simulink model "softmax_int"  (R2024b)
settings: Solver=FixedStepDiscrete  StartTime=0.0  StopTime=20.0  RelTol=1e-3
InitFcn:
  | % Define a random matrix size between 3 and 10
  | n =6;
  | 
  | fprintf('Size of matrix A: n = %d\n', n);
libraries: simulink x1
settings Model: DataTypeOverride=Off  Creator=valen  LastModifiedBy=valen
settings SolverCC: AlgebraicLoopSolver=TrustRegion
settings DataIOCC: LimitDataPoints=on  SaveOutput=off  SaveTime=off
settings OptimizationCC: BlockReduction=off  ConditionallyExecuteInputs=off  DefaultParameterBehavior=Inlined  LifeSpan=inf
settings DebuggingCC: AlgebraicLoopMsg=error  SingleTaskRateTransMsg=error  UnconnectedInputMsg=warning  UnconnectedOutputMsg=warning  UnconnectedLineMsg=warning  AllowSymbolicDim=off  StrictBusMsg=ErrorOnBusTreatedAsVector  SFUnexpectedBacktrackingDiag=warning  SFNoUnconditionalDefaultTransitionDiag=warning  SFExecutionAtInitializationDiag=none  ArithmeticOperatorsInVariantConditions=warning
settings HardwareCC: ProdBitPerPointer=32  ProdBitPerSizeT=32  ProdBitPerPtrDiffT=32  ProdLargestAtomicFloat=None  ProdIntDivRoundTo=Undefined  ProdEndianess=Unspecified  ProdWordSize=32  ProdHWDeviceType=ASIC/FPGA->ASIC/FPGA  ProdEqTarget=off
settings ModelReferenceCC: EnableRefExpFcnMdlSchedulingChecks=on
settings SFSimCC: SimUseLocalCustomCode=off  CustomCodeUndefinedFunction=UseInterfaceOnly
settings RTWCC: RTWUseLocalCustomCode=off  GPUComputeCapability=3.5
settings CodeAppCC: StateflowObjectComments=on
settings GRTTargetCC: TargetLangStandard=C89/C90 (ANSI)
settings ConfigComp: CovScope=ReferencedModels  CovMetricSettings=dw  CovSaveCumulativeToWorkspaceVar=on  CovSaveSingleToWorkspaceVar=on  CovExternalEMLEnable=off  CovSFcnEnable=off

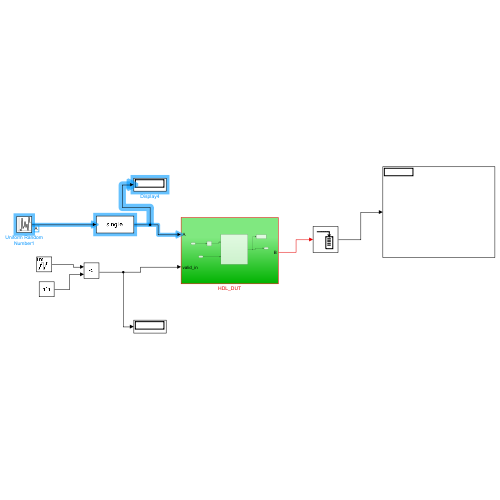
[thumbnail: Simulink's stored preview of the top-level diagram]
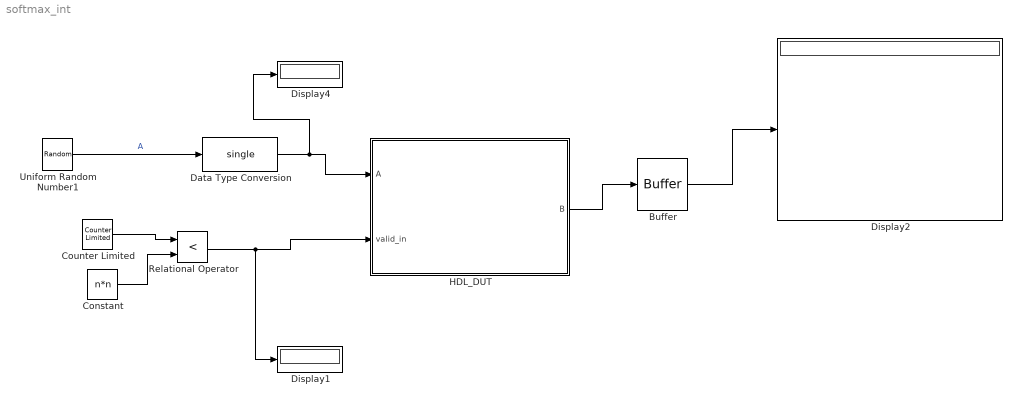
== system softmax_int ==
  Buffer : Buffer  N=2*n*n  OutputFrames=off
  Constant : Constant  Value=n*n
  Counter Limited : simulink/Sources/Counter Limited  uplimit=n*(n+1)  tsamp=-1
  Data Type Conversion : DataTypeConversion  OutDataTypeStr=single  SaturateOnIntegerOverflow=off  RndMeth=Floor
  Display1 : Display
  Display2 : Display
  Display4 : Display
  HDL_DUT : Subsystem
  Relational Operator : RelationalOperator  Operator=<  OutDataTypeStr=boolean  RndMeth=Simplest  InputSameDT=off
  Uniform Random Number1 : UniformRandomNumber  Minimum=0  Maximum=5  Seed=n  SampleTime=10/(n*n+1)
  wires:
  HDL_DUT/1(B) -> Buffer/1
  Uniform Random Number1/1 -> Data Type Conversion/1  "A"
  Buffer/1 -> Display2/1
  Data Type Conversion/1 -> Display4/1, HDL_DUT/1(A)
  Counter Limited/1 -> Relational Operator/1
  Constant/1 -> Relational Operator/2
  Relational Operator/1 -> Display1/1, HDL_DUT/2(valid_in)

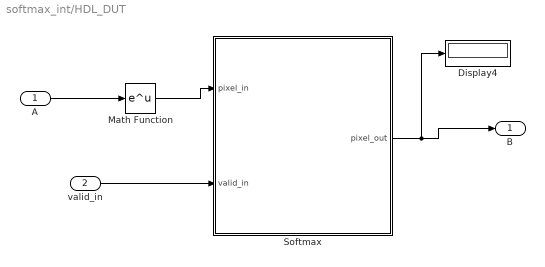
== system softmax_int/HDL_DUT ==
  A : Inport
  valid_in : Inport  Port=2
  Display4 : Display
  Math Function : Math  SignedPower=on  RndMeth=Zero
  Softmax : MATLAB Function  TreatAsAtomicUnit=on
  B : Outport  VectorParamsAs1DForOutWhenUnconnected=off
  wires:
  A/1 -> Math Function/1
  Softmax/1(pixel_out) -> Display4/1, B/1
  valid_in/1 -> Softmax/2(valid_in)
  Math Function/1 -> Softmax/1(pixel_in)

== matlab function softmax_int/HDL_DUT/Softmax ==
  data: pixel_in input; pixel_out output; valid_in input
function pixel_out  = hardware_softmax(pixel_in, valid_in)
    WIDTH = 6;
    TOTAL_PIXELS = WIDTH * WIDTH;
    
    % Registres persistants (Hardware)
    persistent buffer sum_values count state inv_sum;
    if isempty(state)
        buffer = zeros(1, 100, 'single'); % RAM de stockage temporaire
        sum_values = single(0);
        inv_sum = single(0);
        count = int32(1);
        state = int32(0); % 0: Accumulation, 1: Calcul Inverse, 2: Stream Sortie
    end
    
    % Signaux de contrôle par défaut
    pixel_out = single(0);
    valid_out = false;
    
    switch state
        case 0 % --- PASSE 1 : ACCUMULATION & STOCKAGE ---
            if valid_in
                % 2. Stockage dans la mémoire tampon
                buffer(count) = single(pixel_in);
                
                if count == TOTAL_PIXELS
                    count = int32(1);
                    state = int32(1); % Matrice reçue -> Passe à l'étape suivante
                else
                    count = count + 1;
                end
            end
            
        case 1 % --- ÉTAPE INTERMÉDIAIRE : L'INVERSE (1 cycle ou + selon pipeline) ---
            % On calcule l'inverse une seule fois pour éviter les divisions répétées
            % On calcule la somme de tout le buffer d'un seul coup. 
            % HDL Coder va créer un arbre d'additionneurs parallélisé qu'il PEUT pipeliner, 
            % car il n'y a plus de boucle de rétroaction (Feedback) d'un cycle sur l'autre !
            sum_values = sum(buffer);

            inv_sum = single(1) / sum_values; 
            state = int32(2); 
            
        case 2 % --- PASSE 2 : NORMALISATION EN STREAM ---
            % On recrache les pixels un par un en multipliant par l'inverse
            pixel_out = buffer(count) * inv_sum;
           
            if count == TOTAL_PIXELS
                % Réinitialisation pour la matrice suivante
                count = int32(1);
                sum_values = single(0);
                state = int32(0); 
            else
                count = count + 1;
            end
    end
end
